simulink model "DC_DC_G13_sim_L3"  (R2024b)
settings: Solver=ode23tb  StartTime=0.0  StopTime=0.04  MaxStep=1/fpwm/200  RelTol=1e-3
undefined symbols (not defined in the file): Cf, fpwm, IoAVin, Ios, Ki, Kiv, Kp, Kpv, Lf, Po, pr, ri, Rmax, U, ucmax, Vo
libraries: spsSeriesRLCBranchLib x6, spsCurrentMeasurementLib x3, spsMeanLib x3, spsVoltageMeasurementLib x3, spsBreakerLib x2, spsControlledCurrentSourceLib x2, spsDiodeLib x1, simulink x1, spsMosfetLib x1, spsDCVoltageSourceLib x1, sps_lib x1
settings Model: Creator=Martinha  LastModifiedBy=franc

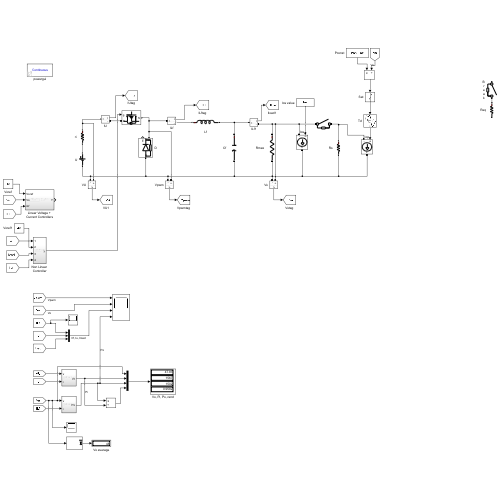
[thumbnail: Simulink's stored preview of the top-level diagram]
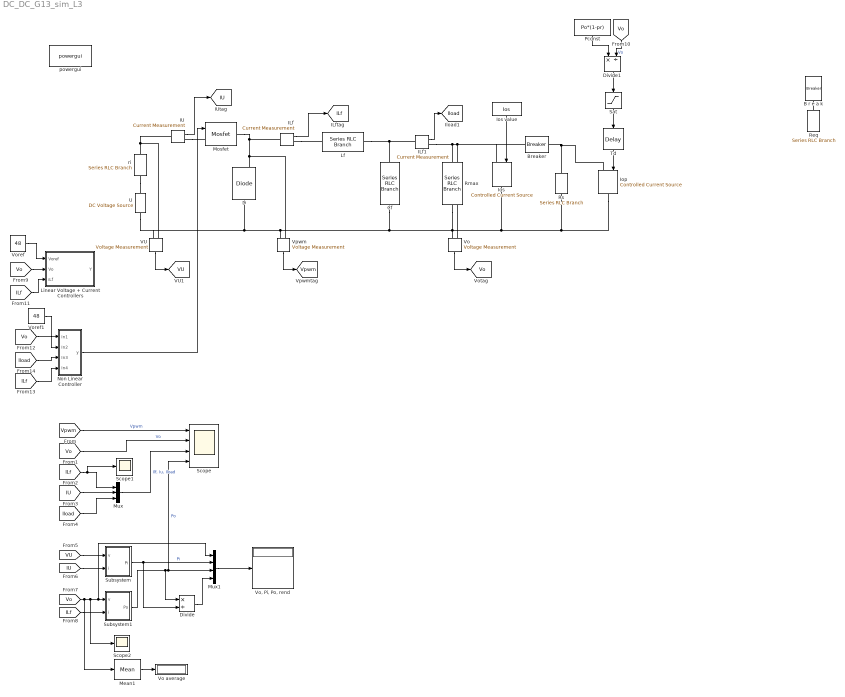
== system DC_DC_G13_sim_L3 ==
  B r e a k : spsBreakerLib/Breaker  InitialState=0  SwitchingTimes=[0.02]  External=off  BreakerResistance=0.01  SnubberResistance=Rs  SnubberCapacitance=Cs  Measurements=None  MoreParameters=on  NoBreakLoop=off
  Breaker : spsBreakerLib/Breaker  InitialState=0  SwitchingTimes=[0.02]  External=off  BreakerResistance=0.01  SnubberResistance=Rs  SnubberCapacitance=Cs  Measurements=None  MoreParameters=on  NoBreakLoop=off
  Cf : spsSeriesRLCBranchLib/Series RLC Branch  LConnTagsString=__new0  RConnTagsString=__new0  BranchType=C  Resistance=1  Inductance=1e-3  SetiL0=off  InitialCurrent=0  Capacitance=Cf  Setx0=on  InitialVoltage=48  Measurements=None
  D : spsDiodeLib/Diode  Ron=Ron  Lon=0  Vf=Vd  IC=0  UseSnubber=0  Rs=Rs  Cs=Cs  Measurements=on
  Divide : Product  Inputs=*/
  Divide1 : Product  Inputs=*/
  ILf : spsCurrentMeasurementLib/Current Measurement  PhasorSimulation=off  OutputType=Complex  PSBequivalent=0
  ILf1 : spsCurrentMeasurementLib/Current Measurement  PhasorSimulation=off  OutputType=Complex  PSBequivalent=0
  IU : spsCurrentMeasurementLib/Current Measurement  PhasorSimulation=off  OutputType=Complex  PSBequivalent=0
  Iop : spsControlledCurrentSourceLib/Controlled Current Source  Initialize=on  Source_Type=DC  Amplitude=0  Phase=0  Frequency=0  Measurements=Current
  Ios : spsControlledCurrentSourceLib/Controlled Current Source  Initialize=on  Source_Type=DC  Amplitude=0  Phase=0  Frequency=0  Measurements=Current
  Ios value : Constant  Value=Ios
  Lf : spsSeriesRLCBranchLib/Series RLC Branch  LConnTagsString=__new0  RConnTagsString=__new0  BranchType=L  Resistance=1  Inductance=Lf  SetiL0=off  InitialCurrent=0  Capacitance=1e-6  Setx0=off  InitialVoltage=0  Measurements=None
  Linear Voltage + Current Controllers : Subsystem
  Mean1 : spsMeanLib/Mean  Freq=fpwm/10  Vinit=110  Ts=0
  Mosfet : spsMosfetLib/Mosfet  Ron=Ron  Lon=0  Rd=Rdson  Vfd=Vd  IC=0  Rs=Rs  Cs=Cs  Measurements=off
  Mux : Mux  Inputs=3
  Mux1 : Mux
  Non Linear Controller : Subsystem
  Pconst : Constant  Value=Po*(1-pr)
  Req : spsSeriesRLCBranchLib/Series RLC Branch  LConnTagsString=__new0  RConnTagsString=__new0  BranchType=R  Resistance=Rmax/14  Inductance=1e-3  SetiL0=off  InitialCurrent=0  Capacitance=1e-6  Setx0=off  InitialVoltage=0  Measurements=None
  Rmax : spsSeriesRLCBranchLib/Series RLC Branch  LConnTagsString=__new0  RConnTagsString=__new0  BranchType=R  Resistance=Vo^2/(Po*pr)  Inductance=1e-3  SetiL0=off  InitialCurrent=0  Capacitance=1e-6  Setx0=off  InitialVoltage=0  Measurements=None
  Rs : spsSeriesRLCBranchLib/Series RLC Branch  LConnTagsString=__new0  RConnTagsString=__new0  BranchType=R  Resistance=100*Rmax  Inductance=1e-3  SetiL0=off  InitialCurrent=0  Capacitance=1e-6  Setx0=off  InitialVoltage=0  Measurements=None
  Sat : Saturate  UpperLimit=100  LowerLimit=0
  Scope : Scope  NumInputPorts=4
  Scope1 : Scope
  Scope2 : Scope
  Subsystem : Subsystem
  Subsystem1 : Subsystem
  Td : TransportDelay  DelayTime=1/(2*fpwm)
  U : spsDCVoltageSourceLib/DC Voltage Source  Amplitude=U  Measurements=None
  VU : spsVoltageMeasurementLib/Voltage Measurement  PhasorSimulation=off  OutputType=Complex  PSBequivalent=0
  Vo : spsVoltageMeasurementLib/Voltage Measurement  PhasorSimulation=off  OutputType=Complex  PSBequivalent=0
  Vo average : Display
  "Vo, Pi, Po, rend" : Display
  Voref : Constant  Value=48
  Voref1 : Constant  Value=48
  Vpwm : spsVoltageMeasurementLib/Voltage Measurement  PhasorSimulation=off  OutputType=Complex  PSBequivalent=0
  powergui : sps_lib/powergui  Priority=1  SimulationMode=Continuous  SampleTime=50e-6  frequency=60  Iterations=50  frequencyindice=0  Pbase=100e6  ErrMax=1e-4  UnitsV=kV  UnitsW=MW  buscounter=0  FunctionMessages=off  echomessages=off  EnableUseOfTLC=off  CurrentSourceSwitches=off  DisableSnubberDevices=off  DisableRonSwitches=off  DisableVfSwitches=off  DisplayEquations=off  AutomaticDiscreteSolvers=off  SolverType=Tustin/Backward Euler (TBE)  Interpol=off  ExternalGateDelay=off  methode=off  Ts=100  x0status=blocks  SPID=on  SwTol=0  HookPort=off  NonlinearTolerance=1e-4  nMaxIteration=100  ContinueOnMaxIteration=off  RestoreLinks=warning  ResistiveCurrentMeasurement=off  Frange=[0:2:500]  Ylog=off  Xlog=on  ShowGrid=off  save=off  variable=ZData  structure=0  ZoomFFT=off  StartTime=0.0  cycles=1  DisplayStyle=1  fundamental=60  FreqAxis=off  MaxFrequency=1000  frequencyindicesteady=1  RmsSteady=1  display=off
  ri : spsSeriesRLCBranchLib/Series RLC Branch  LConnTagsString=__new0  RConnTagsString=__new0  BranchType=R  Resistance=ri  Inductance=1e-3  SetiL0=off  InitialCurrent=0  Capacitance=1e-6  Setx0=off  InitialVoltage=0  Measurements=None
  tag scope: ILf=global, IU=global, Iload=global, VU=global, Vo=global, Vpwm=global
  wires:
  IU/1 -> [IU]
  VU/1 -> [VU]
  Vpwm/1 -> [Vpwm]
  Vo/1 -> [Vo]
  ILf1/1 -> [Iload]
  ILf/1 -> [ILf]
  [ILf] -> Scope1/1, Mux/1
  [IU] -> Mux/2
  [Iload] -> Mux/3
  [VU] -> Subsystem/1(v)
  [IU] -> Subsystem/2(i)
  [ILf] -> Subsystem1/2(i)
  Subsystem/1(Pi) -> Divide/2, Mux1/2  "Pi"
  Subsystem1/1(Po) -> Scope/4, Mux1/3, Divide/1  "Po"
  Mux1/1 -> "Vo, Pi, Po, rend"/1
  Divide/1 -> Mux1/4
  [Vpwm] -> Scope/1  "Vpwm"
  Mux/1 -> Scope/3  "Ilf, Iu, Iload"
  [Vo] -> Mean1/1, Scope2/1, Mux1/1, Subsystem1/1(v)
  [Vo] -> Scope/2  "Vo"
  Td/1 -> Iop/1
  Sat/1 -> Td/1
  Divide1/1 -> Sat/1
  Pconst/1 -> Divide1/1
  [Vo] -> Divide1/2  "Vo"
  Ios value/1 -> Ios/1
  Voref/1 -> Linear Voltage + Current Controllers/1(Voref)
  [Vo] -> Linear Voltage + Current Controllers/2(Vo)
  [ILf] -> Linear Voltage + Current Controllers/3(iLf)
  Mean1/1 -> Vo average/1
  Voref1/1 -> Non Linear Controller/1(In1)
  [Vo] -> Non Linear Controller/2(In2)
  [ILf] -> Non Linear Controller/4(In4)
  [Iload] -> Non Linear Controller/3(In3)
  Non Linear Controller/1(y) -> Mosfet/1
  connections:
  Lf/RConn1 -- ILf1/LConn1 -- Cf/LConn1
  Mosfet/RConn1 -- Vpwm/LConn1 -- D/RConn1 -- ILf/LConn1
  IU/RConn1 -- Mosfet/LConn1
  ri/RConn1 -- U/RConn1
  ri/LConn1 -- VU/LConn1 -- IU/LConn1
  ILf/RConn1 -- Lf/LConn1
  Rmax/LConn1 -- Ios/LConn1 -- Breaker/LConn1 -- Vo/LConn1 -- ILf1/RConn1
  Rs/LConn1 -- Iop/LConn1 -- Breaker/RConn1
  Rs/RConn1 -- Ios/RConn1 -- Vo/LConn2 -- Rmax/RConn1 -- U/LConn1 -- VU/LConn2 -- D/LConn1 -- Vpwm/LConn2 -- Cf/RConn1 -- Iop/RConn1
  Req/LConn1 -- B r e a k/RConn1

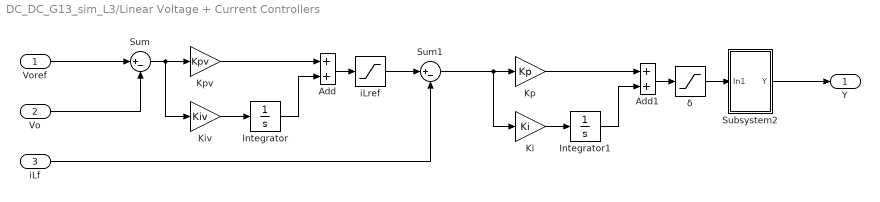
== system DC_DC_G13_sim_L3/Linear Voltage + Current Controllers ==
  Voref : Inport
  Vo : Inport  Port=2
  iLf : Inport  Port=3
  Add : Sum
  Add1 : Sum
  Integrator : Integrator  LimitOutput=on  UpperSaturationLimit=60  LowerSaturationLimit=-60
  Integrator1 : Integrator  LimitOutput=on  UpperSaturationLimit=1  LowerSaturationLimit=-1
  Ki : Gain  Gain=Ki
  Kiv : Gain  Gain=Kiv
  Kp : Gain  Gain=Kp
  Kpv : Gain  Gain=Kpv
  Subsystem2 : Subsystem
  Sum : Sum  Inputs=|+-
  Sum1 : Sum  Inputs=|+-
  iLref : Saturate  UpperLimit=60  LowerLimit=0
  δ : Saturate  UpperLimit=0.99  LowerLimit=0.01
  Y : Outport
  wires:
  Voref/1 -> Sum/1
  Sum1/1 -> Ki/1, Kp/1
  Subsystem2/1(Y) -> Y/1
  Integrator/1 -> Add/2
  Add1/1 -> δ/1
  Integrator1/1 -> Add1/2
  Kpv/1 -> Add/1
  iLf/1 -> Sum1/2
  Add/1 -> iLref/1
  Sum/1 -> Kiv/1, Kpv/1
  Kp/1 -> Add1/1
  Ki/1 -> Integrator1/1
  δ/1 -> Subsystem2/1(In1)
  Kiv/1 -> Integrator/1
  iLref/1 -> Sum1/1
  Vo/1 -> Sum/2

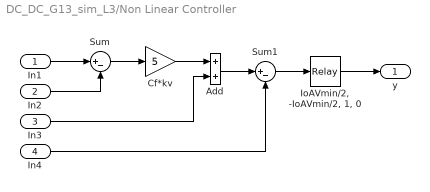
== system DC_DC_G13_sim_L3/Non Linear Controller ==
  In1 : Inport
  In2 : Inport  Port=2
  In3 : Inport  Port=3
  In4 : Inport  Port=4
  Add : Sum
  Cf*kv : Gain  Gain=5
  "IoAVmin/2, -IoAVmin/2, 1, 0" : Relay  OnSwitchValue=IoAVin  OffSwitchValue=-IoAVin
  Sum : Sum  Inputs=|+-
  Sum1 : Sum  Inputs=|+-
  y : Outport
  wires:
  In4/1 -> Sum1/2
  In3/1 -> Add/2
  In1/1 -> Sum/1
  "IoAVmin/2, -IoAVmin/2, 1, 0"/1 -> y/1
  Sum1/1 -> "IoAVmin/2, -IoAVmin/2, 1, 0"/1
  Add/1 -> Sum1/1
  Sum/1 -> Cf*kv/1
  Cf*kv/1 -> Add/1
  In2/1 -> Sum/2

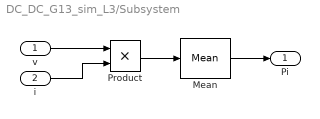
== system DC_DC_G13_sim_L3/Subsystem ==
  v : Inport
  i : Inport  Port=2
  Mean : spsMeanLib/Mean  Freq=fpwm/10  Vinit=110  Ts=0
  Product : Product
  Pi : Outport
  wires:
  Mean/1 -> Pi/1
  i/1 -> Product/2
  v/1 -> Product/1
  Product/1 -> Mean/1

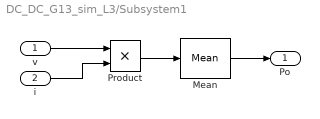
== system DC_DC_G13_sim_L3/Subsystem1 ==
  v : Inport
  i : Inport  Port=2
  Mean : spsMeanLib/Mean  Freq=fpwm/10  Vinit=110  Ts=0
  Product : Product
  Po : Outport
  wires:
  Mean/1 -> Po/1
  i/1 -> Product/2
  v/1 -> Product/1
  Product/1 -> Mean/1

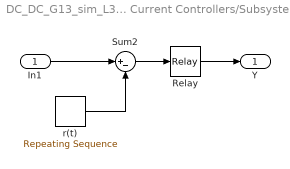
== system DC_DC_G13_sim_L3/Linear Voltage + Current Controllers/Subsystem2 ==
  In1 : Inport
  Relay : Relay  OnSwitchValue=0.01  OffSwitchValue=-0.01
  Sum2 : Sum  Inputs=|+-
  "r(t) " : simulink/Sources/Repeating Sequence  rep_seq_t=[0 1/fpwm]  rep_seq_y=[0 ucmax]
  Y : Outport
  wires:
  "r(t) "/1 -> Sum2/2
  Relay/1 -> Y/1
  In1/1 -> Sum2/1
  Sum2/1 -> Relay/1
